simulink model "Lab06"  (Simulink 7.4)
settings: Solver=ode45  StartTime=0.0  StopTime=10.0  RelTol=1e-3
settings Model: Creator=AshfaqAhmad  LastModifiedBy=AshfaqAhmad

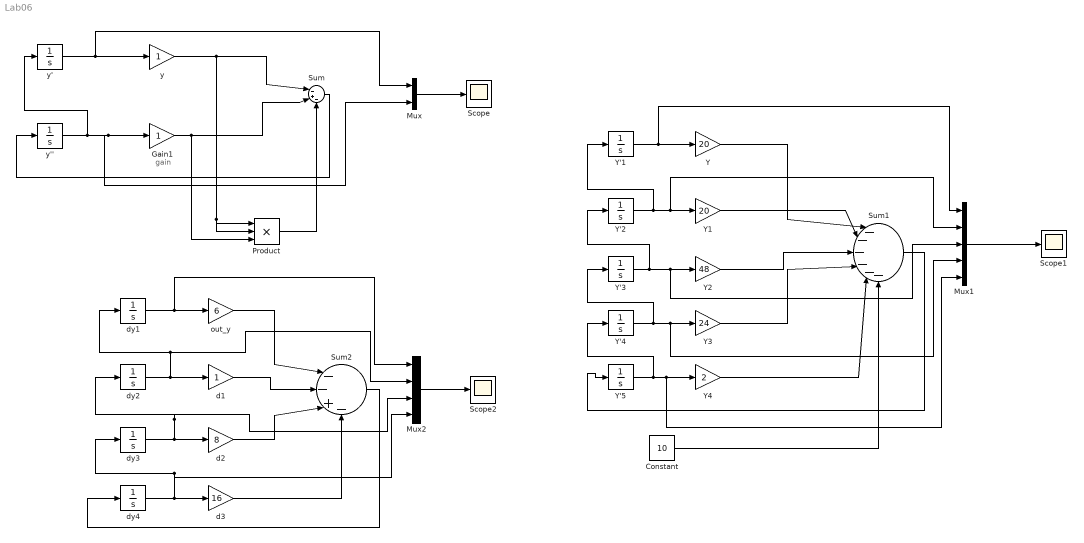
== system Lab06 ==
  note: gain
  Constant : Constant  Value=10  OutDataType=fixdt(1, 16)  OutScaling=2^0
  Gain1 : Gain  ParameterDataType=fixdt(1, 16)  ParameterScaling=2^0  OutDataType=fixdt(1, 16)  OutScaling=2^0
  Mux : Mux  Inputs=2
  Mux1 : Mux  Inputs=5
  Mux2 : Mux
  Product : Product  Inputs=3  OutDataType=fixdt(1, 16)  OutScaling=2^0  RndMeth=Zero
  Scope : Scope
  Scope1 : Scope
  Scope2 : Scope
      settings: SaveName=ScopeData2
  Sum : Sum  Inputs=|-+-  OutDataType=fixdt(1, 16)  OutScaling=2^0
  Sum1 : Sum  Inputs=|------  OutDataType=fixdt(1, 16)  OutScaling=2^0
  Sum2 : Sum  Inputs=|--+-  OutDataType=fixdt(1, 16)  OutScaling=2^0
  Y : Gain  Gain=20  ParameterDataType=fixdt(1, 16)  ParameterScaling=2^0  OutDataType=fixdt(1, 16)  OutScaling=2^0
  Y'1 : Integrator  InitialCondition=2
  Y'2 : Integrator  InitialCondition=5
  Y'3 : Integrator  InitialCondition=10
  Y'4 : Integrator  InitialCondition=-4
  Y'5 : Integrator  InitialCondition=-7
  Y1 : Gain  Gain=20  ParameterDataType=fixdt(1, 16)  ParameterScaling=2^0  OutDataType=fixdt(1, 16)  OutScaling=2^0
  Y2 : Gain  Gain=48  ParameterDataType=fixdt(1, 16)  ParameterScaling=2^0  OutDataType=fixdt(1, 16)  OutScaling=2^0
  Y3 : Gain  Gain=24  ParameterDataType=fixdt(1, 16)  ParameterScaling=2^0  OutDataType=fixdt(1, 16)  OutScaling=2^0
  Y4 : Gain  Gain=2  ParameterDataType=fixdt(1, 16)  ParameterScaling=2^0  OutDataType=fixdt(1, 16)  OutScaling=2^0
  d1 : Gain  ParameterDataType=fixdt(1, 16)  ParameterScaling=2^0  OutDataType=fixdt(1, 16)  OutScaling=2^0
  d2 : Gain  Gain=8  ParameterDataType=fixdt(1, 16)  ParameterScaling=2^0  OutDataType=fixdt(1, 16)  OutScaling=2^0
  d3 : Gain  Gain=16  ParameterDataType=fixdt(1, 16)  ParameterScaling=2^0  OutDataType=fixdt(1, 16)  OutScaling=2^0
  dy1 : Integrator  InitialCondition=4
  dy2 : Integrator
  dy3 : Integrator  InitialCondition=-6
  dy4 : Integrator  InitialCondition=2
  out_y : Gain  Gain=6  ParameterDataType=fixdt(1, 16)  ParameterScaling=2^0  OutDataType=fixdt(1, 16)  OutScaling=2^0
  y : Gain  ParameterDataType=fixdt(1, 16)  ParameterScaling=2^0  OutDataType=fixdt(1, 16)  OutScaling=2^0
  y' : Integrator
  y'' : Integrator  InitialCondition=12
  wires:
  y'/1 -> y/1, Mux/1
  y''/1 -> Gain1/1, Mux/2, y'/1
  Sum/1 -> y''/1
  y/1 -> Sum/1, Product/1, Product/2
  Mux/1 -> Scope/1
  Gain1/1 -> Sum/2, Product/3
  Product/1 -> Sum/3
  Y'1/1 -> Y/1, Mux1/1
  Y'2/1 -> Y'1/1, Y1/1, Mux1/2
  Y'3/1 -> Y'2/1, Y2/1, Mux1/3
  Y'4/1 -> Y'3/1, Y3/1, Mux1/4
  Y'5/1 -> Y'4/1, Y4/1, Mux1/5
  Mux1/1 -> Scope1/1
  Y4/1 -> Sum1/5
  Y3/1 -> Sum1/4
  Y2/1 -> Sum1/3
  Y1/1 -> Sum1/2
  Y/1 -> Sum1/1
  Constant/1 -> Sum1/6
  Sum1/1 -> Y'5/1
  dy1/1 -> out_y/1, Mux2/1
  dy2/1 -> d1/1, dy1/1, Mux2/2
  dy3/1 -> d2/1, dy2/1, Mux2/3
  dy4/1 -> dy3/1, Mux2/4, d3/1
  d3/1 -> Sum2/4
  d1/1 -> Sum2/2
  out_y/1 -> Sum2/1
  Sum2/1 -> dy4/1
  Mux2/1 -> Scope2/1
  d2/1 -> Sum2/3
